simulink model "simulation_Hippocampus_CDC"  (R2021a)
settings: Solver=ode45  StartTime=0.0  StopTime=50  FixedStep=0.00001  MaxStep=0.1  MinStep=0.00001  RelTol=1e-5
libraries: simulink x3
(part 1 of 2)
settings Model: Creator=ch  LastModifiedBy=sf
settings SolverCC: MaxConsecutiveZCs=100000  ZeroCrossAlgorithm=Adaptive  AlgebraicLoopSolver=TrustRegion  PositivePriorityOrder=on  AutoInsertRateTranBlk=on
settings DebuggingCC: MaskedZcDiagnostic=none  IgnoredZcDiagnostic=none  SFMachineParentedDataDiag=warning  ArithmeticOperatorsInVariantConditions=warning
settings SFSimCC: CustomCodeUndefinedFunction=UseInterfaceOnly

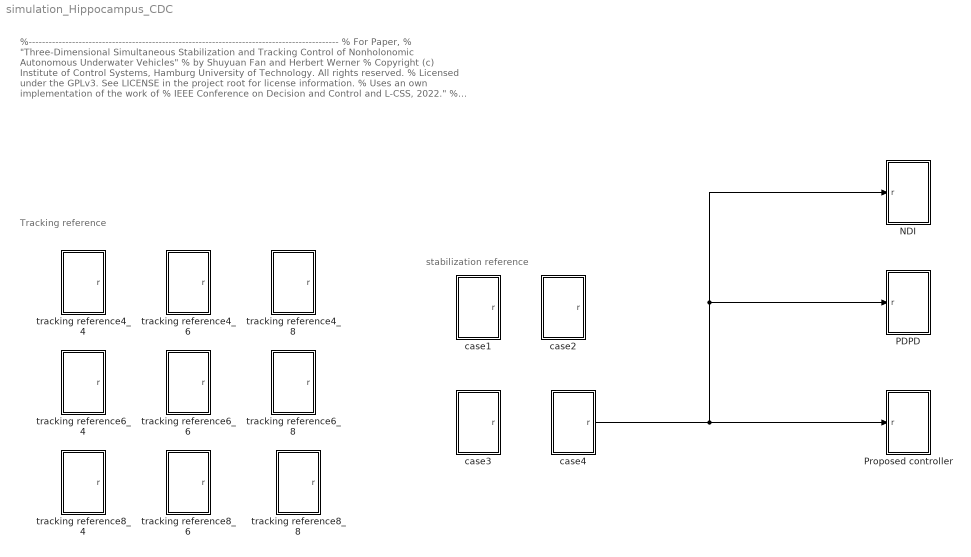
== system simulation_Hippocampus_CDC ==
  note: %---------------------------------------------------------------------------------------------
      | % For Paper,
      | % "Three-Dimensional Simultaneous Stabilization and Tracking Control of Nonholonomic Autonomous Underwater Vehicles"
      | % by Shuyuan Fan and Herbert Werner
      | % Copyright (c) Institute of Control Systems, Hamburg University of Technology. All rights reserved.
      | % Licensed under the GPLv3. See LICENSE in the project root for license information.
      | % Uses an own implementation of the work of
      | % IEEE Conference on Decision and Control and L-CSS, 2022."
      | % Author(s): Shuyuan Fan
      | %--------------------------------------------------------------------------------------------
  note: Tracking reference
  note: stabilization reference
  NDI : Subsystem
  PDPD : Subsystem
  Proposed controller : Subsystem
  case1 : Subsystem
  case2 : Subsystem
  case3 : Subsystem
  case4 : Subsystem
  tracking reference4_4 : Subsystem
  tracking reference4_6 : Subsystem
  tracking reference4_8 : Subsystem
  tracking reference6_4 : Subsystem
  tracking reference6_6 : Subsystem
  tracking reference6_8 : Subsystem
  tracking reference8_4 : Subsystem
  tracking reference8_6 : Subsystem
  tracking reference8_8 : Subsystem
  wires:
  case4/1(r) -> NDI/1(r), PDPD/1(r), Proposed controller/1(r)

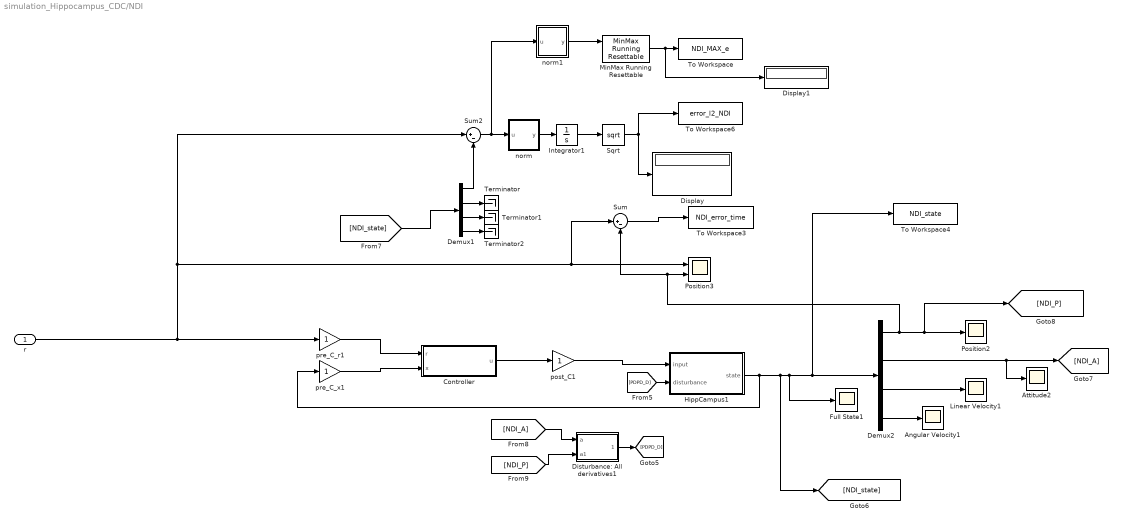
== system simulation_Hippocampus_CDC/NDI ==
  r : Inport
  Angular Velocity1 : Scope
  Attitude2 : Scope
  Controller : Subsystem
  Demux1 : Demux  Outputs=[3 3 3 3]
  Demux2 : Demux  Outputs=[3 3 3 3]
  Display : Display
  Display1 : Display
  Disturbance: All derivatives1 : Subsystem
  Full State1 : Scope
  HippCampus1 : Subsystem
  Integrator1 : Integrator
  Linear Velocity1 : Scope
  MinMax Running Resettable : simulink/Math Operations/MinMax Running Resettable  Function=max  vinit=0.0
  Position2 : Scope
  Position3 : Scope  NumInputPorts=2
  Sqrt : Sqrt  SaturateOnIntegerOverflow=on
  Sum : Sum  Inputs=|+-
  Sum2 : Sum  Inputs=|+-
  Terminator : Terminator
  Terminator1 : Terminator
  Terminator2 : Terminator
  To Workspace : ToWorkspace  VariableName=NDI_MAX_e  SaveFormat=Timeseries  SampleTime=-1
  To Workspace3 : ToWorkspace  VariableName=NDI_error_time  SaveFormat=Timeseries  SampleTime=-1
  To Workspace4 : ToWorkspace  VariableName=NDI_state  SaveFormat=Timeseries  SampleTime=-1
  To Workspace6 : ToWorkspace  VariableName=error_l2_NDI  SaveFormat=Timeseries  SampleTime=-1
      settings: MaxDataPoints=1
  norm : MATLAB Function  TreatAsAtomicUnit=on
  norm1 : MATLAB Function  TreatAsAtomicUnit=on
  post_C1 : Gain
  pre_C_r1 : Gain
  pre_C_x1 : Gain
  wires:
  Controller/1(u) -> post_C1/1
  [PDPD_D] -> HippCampus1/2(disturbance)
  Demux2/2 -> Attitude2/1, [NDI_A]
  HippCampus1/1(state) -> To Workspace4/1, Demux2/1, Full State1/1, [NDI_state], pre_C_x1/1
  pre_C_r1/1 -> Controller/1(r)
  Demux2/3 -> Linear Velocity1/1
  post_C1/1 -> HippCampus1/1(input)
  Disturbance: All derivatives1/1(disturbance) -> [PDPD_D]
  [NDI_P] -> Disturbance: All derivatives1/2(a1)
  pre_C_x1/1 -> Controller/2(x)
  Demux2/4 -> Angular Velocity1/1
  [NDI_A] -> Disturbance: All derivatives1/1(a)
  [NDI_state] -> Demux1/1
  Demux1/3 -> Terminator1/1
  Integrator1/1 -> Sqrt/1
  norm/1(y) -> Integrator1/1
  Demux1/2 -> Terminator/1
  Demux1/1 -> Sum2/2
  Demux1/4 -> Terminator2/1
  Sqrt/1 -> To Workspace6/1, Display/1
  Sum2/1 -> norm1/1(u), norm/1(u)
  norm1/1(y) -> MinMax Running Resettable/1
  MinMax Running Resettable/1 -> Display1/1, To Workspace/1
  Sum/1 -> To Workspace3/1
  r/1 -> Sum/1, Position3/1, Sum2/1, pre_C_r1/1
  Demux2/1 -> [NDI_P], Position2/1, Sum/2, Position3/2

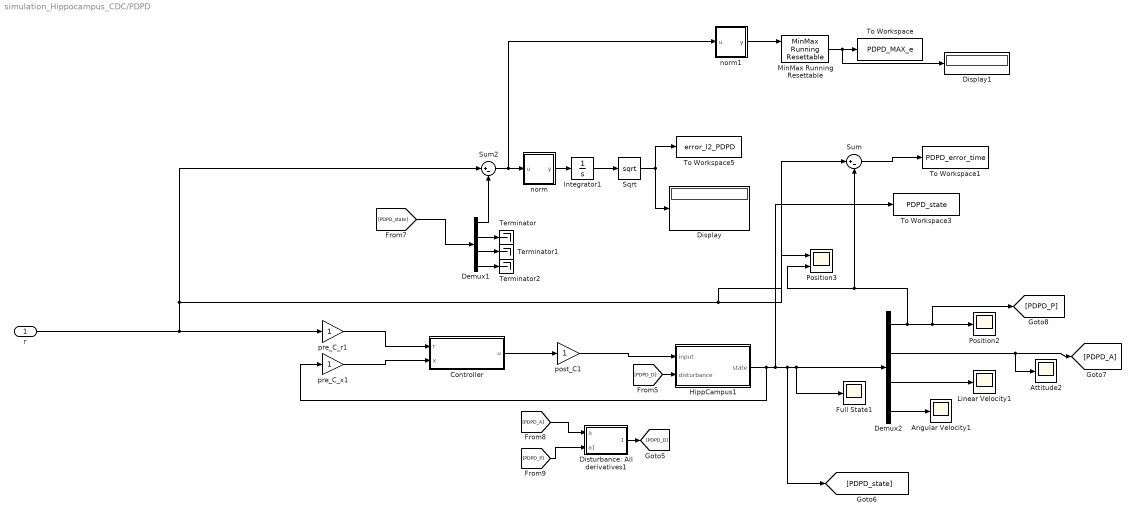
== system simulation_Hippocampus_CDC/PDPD ==
  r : Inport
  Angular Velocity1 : Scope
  Attitude2 : Scope
  Controller : Subsystem
  Demux1 : Demux  Outputs=[3 3 3 3]
  Demux2 : Demux  Outputs=[3 3 3 3]
  Display : Display
  Display1 : Display
  Disturbance: All derivatives1 : Subsystem
  Full State1 : Scope
  HippCampus1 : Subsystem
  Integrator1 : Integrator
  Linear Velocity1 : Scope
  MinMax Running Resettable : simulink/Math Operations/MinMax Running Resettable  Function=max  vinit=0.0
  Position2 : Scope
  Position3 : Scope  NumInputPorts=2
  Sqrt : Sqrt  SaturateOnIntegerOverflow=on
  Sum : Sum  Inputs=|+-
  Sum2 : Sum  Inputs=|+-
  Terminator : Terminator
  Terminator1 : Terminator
  Terminator2 : Terminator
  To Workspace : ToWorkspace  VariableName=PDPD_MAX_e  SaveFormat=Timeseries  SampleTime=-1
  To Workspace1 : ToWorkspace  VariableName=PDPD_error_time  SaveFormat=Timeseries  SampleTime=-1
  To Workspace3 : ToWorkspace  VariableName=PDPD_state  SaveFormat=Timeseries  SampleTime=-1
  To Workspace5 : ToWorkspace  VariableName=error_l2_PDPD  SaveFormat=Timeseries  SampleTime=-1
      settings: MaxDataPoints=1
  norm : MATLAB Function  TreatAsAtomicUnit=on
  norm1 : MATLAB Function  TreatAsAtomicUnit=on
  post_C1 : Gain
  pre_C_r1 : Gain
  pre_C_x1 : Gain
  wires:
  [PDPD_D] -> HippCampus1/2(disturbance)
  Demux2/2 -> Attitude2/1, [PDPD_A]
  HippCampus1/1(state) -> Full State1/1, Demux2/1, [PDPD_state], To Workspace3/1, pre_C_x1/1
  pre_C_r1/1 -> Controller/1(r)
  Demux2/3 -> Linear Velocity1/1
  post_C1/1 -> HippCampus1/1(input)
  Disturbance: All derivatives1/1(disturbance) -> [PDPD_D]
  [PDPD_P] -> Disturbance: All derivatives1/2(a1)
  pre_C_x1/1 -> Controller/2(x)
  Demux2/4 -> Angular Velocity1/1
  [PDPD_A] -> Disturbance: All derivatives1/1(a)
  [PDPD_state] -> Demux1/1
  Demux1/3 -> Terminator1/1
  Integrator1/1 -> Sqrt/1
  norm/1(y) -> Integrator1/1
  Demux1/2 -> Terminator/1
  Demux1/1 -> Sum2/2
  Demux1/4 -> Terminator2/1
  Sqrt/1 -> To Workspace5/1, Display/1
  Controller/1(u) -> post_C1/1
  norm1/1(y) -> MinMax Running Resettable/1
  MinMax Running Resettable/1 -> Display1/1, To Workspace/1
  Sum2/1 -> norm1/1(u), norm/1(u)
  Sum/1 -> To Workspace1/1
  r/1 -> Sum/1, Position3/1, Sum2/1, pre_C_r1/1
  Demux2/1 -> [PDPD_P], Position2/1, Sum/2, Position3/2

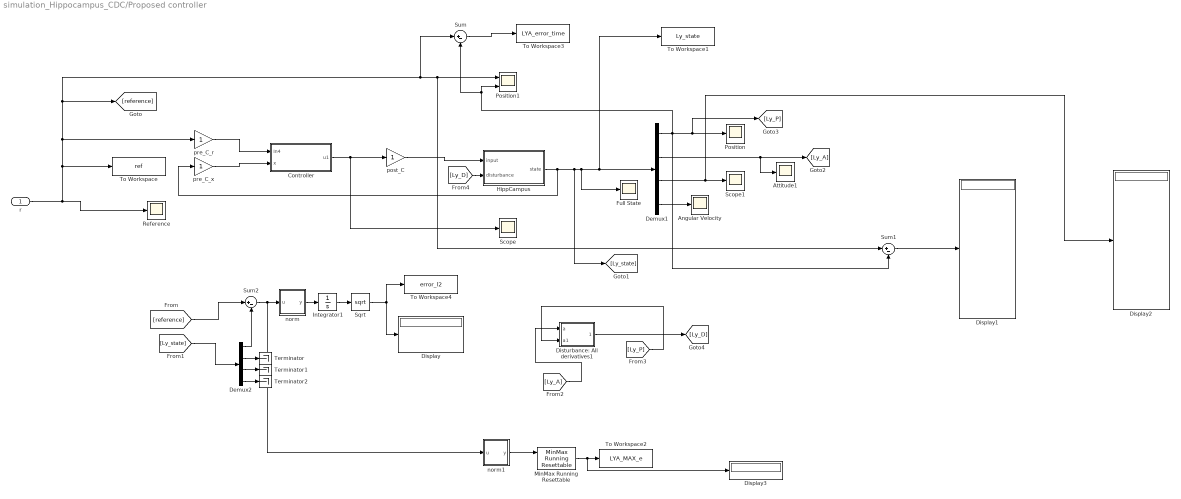
== system simulation_Hippocampus_CDC/Proposed controller ==
  r : Inport
  Angular Velocity : Scope
  Attitude1 : Scope
  Controller : Subsystem
  Demux1 : Demux  Outputs=[3 3 3 3]
  Demux2 : Demux  Outputs=[3 3 3 3]
  Display{,1..3} (4 alike) : Display
  Disturbance: All derivatives1 : Subsystem
  Full State : Scope
  HippCampus : Subsystem
  Integrator1 : Integrator
  MinMax Running Resettable : simulink/Math Operations/MinMax Running Resettable  Function=max  vinit=0.0
  Position : Scope
  Position1 : Scope  NumInputPorts=2
  Reference : Scope
  Scope : Scope
  Scope1 : Scope
  Sqrt : Sqrt  SaturateOnIntegerOverflow=on
  Sum : Sum  Inputs=|+-
  Sum1 : Sum  Inputs=|+-
  Sum2 : Sum  Inputs=|+-
  Terminator : Terminator
  Terminator1 : Terminator
  Terminator2 : Terminator
  To Workspace : ToWorkspace  VariableName=ref  SaveFormat=Timeseries  SampleTime=-1
  To Workspace1 : ToWorkspace  VariableName=Ly_state  SaveFormat=Timeseries  SampleTime=-1
  To Workspace2 : ToWorkspace  VariableName=LYA_MAX_e  SaveFormat=Timeseries  SampleTime=-1
  To Workspace3 : ToWorkspace  VariableName=LYA_error_time  SaveFormat=Timeseries  SampleTime=-1
  To Workspace4 : ToWorkspace  VariableName=error_l2  SaveFormat=Timeseries  SampleTime=-1
      settings: MaxDataPoints=1
  norm : MATLAB Function  TreatAsAtomicUnit=on
  norm1 : MATLAB Function  TreatAsAtomicUnit=on
  post_C : Gain
  pre_C_r : Gain
  pre_C_x : Gain
  wires:
  HippCampus/1(state) -> To Workspace1/1, Demux1/1, Full State/1, [Ly_state], pre_C_x/1
  Disturbance: All derivatives1/1(disturbance) -> [Ly_D]
  Demux1/3 -> Scope1/1, Display2/1
  Demux2/3 -> Terminator1/1
  [Ly_state] -> Demux2/1
  Controller/1(u1) -> Scope/1, post_C/1
  [reference] -> Sum2/1
  Demux2/1 -> Sum2/2
  norm/1(y) -> Integrator1/1
  pre_C_x/1 -> Controller/2(x)
  Integrator1/1 -> Sqrt/1
  Sqrt/1 -> To Workspace4/1, Display/1
  Demux1/4 -> Angular Velocity/1
  [Ly_D] -> HippCampus/2(disturbance)
  Demux1/2 -> Attitude1/1, [Ly_A]
  pre_C_r/1 -> Controller/1(In4)
  Demux2/4 -> Terminator2/1
  Demux1/1 -> [Ly_P], Position/1, Sum/2, Position1/2, Sum1/2
  post_C/1 -> HippCampus/1(input)
  [Ly_P] -> Disturbance: All derivatives1/2(a1)
  Demux2/2 -> Terminator/1
  [Ly_A] -> Disturbance: All derivatives1/1(a)
  Sum2/1 -> norm/1(u), norm1/1(u)
  MinMax Running Resettable/1 -> Display3/1, To Workspace2/1
  norm1/1(y) -> MinMax Running Resettable/1
  Sum/1 -> To Workspace3/1
  r/1 -> Sum/1, Sum1/1, Position1/1, [reference], pre_C_r/1, To Workspace/1, Reference/1
  Sum1/1 -> Display1/1

== system simulation_Hippocampus_CDC/case1 ==
  Constant : Constant  Value=1.5
  Constant1 : Constant
  Constant2 : Constant  Value=2
  Mux3 : Mux  Inputs=[1 1 1]
  r : Outport
  wires:
  Constant1/1 -> Mux3/3
  Constant2/1 -> Mux3/1
  Constant/1 -> Mux3/2
  Mux3/1 -> r/1  "r"

== system simulation_Hippocampus_CDC/case2 ==
  Constant : Constant  Value=-1.5
  Constant1 : Constant  Value=-1
  Constant2 : Constant  Value=2
  Mux3 : Mux  Inputs=[1 1 1]
  r : Outport
  wires:
  Constant1/1 -> Mux3/3
  Constant2/1 -> Mux3/1
  Constant/1 -> Mux3/2
  Mux3/1 -> r/1  "r"

== system simulation_Hippocampus_CDC/case3 ==
  Constant : Constant  Value=2
  Constant1 : Constant  Value=-1
  Constant2 : Constant  Value=1.5
  Mux3 : Mux  Inputs=[1 1 1]
  r : Outport
  wires:
  Constant1/1 -> Mux3/3
  Constant2/1 -> Mux3/1
  Constant/1 -> Mux3/2
  Mux3/1 -> r/1  "r"

== system simulation_Hippocampus_CDC/case4 ==
  Constant : Constant  Value=-2
  Constant1 : Constant  Value=1.5
  Constant2 : Constant
  Mux3 : Mux  Inputs=[1 1 1]
  r : Outport
  wires:
  Constant1/1 -> Mux3/3
  Constant2/1 -> Mux3/1
  Constant/1 -> Mux3/2
  Mux3/1 -> r/1  "r"

== system simulation_Hippocampus_CDC/tracking reference4_4 ==
  Clock : Clock
  Cos : Trigonometry
  Cos1 : Trigonometry
  Gain5 : Gain  Gain=0.1
  Gain6 : Gain  Gain=4
  Gain7 : Gain  Gain=4
  Gain8 : Gain  Gain=pi/15
  Gain9 : Gain  Gain=pi/30
  Mux : Mux  Inputs=3
  r : Outport
  wires:
  Gain9/1 -> Cos/1
  Gain6/1 -> Mux/1
  Gain7/1 -> Mux/2
  Cos1/1 -> Gain6/1
  Cos/1 -> Gain7/1
  Mux/1 -> r/1  "r"
  Gain8/1 -> Cos1/1
  Gain5/1 -> Mux/3
  Clock/1 -> Gain5/1, Gain9/1, Gain8/1

== system simulation_Hippocampus_CDC/tracking reference4_6 ==
  Clock : Clock
  Cos : Trigonometry
  Cos1 : Trigonometry
  Gain5 : Gain  Gain=0.1
  Gain6 : Gain  Gain=4
  Gain7 : Gain  Gain=6
  Gain8 : Gain  Gain=pi/15
  Gain9 : Gain  Gain=pi/30
  Mux : Mux  Inputs=3
  r : Outport
  wires:
  Gain9/1 -> Cos/1
  Gain6/1 -> Mux/1
  Gain7/1 -> Mux/2
  Cos1/1 -> Gain6/1
  Cos/1 -> Gain7/1
  Mux/1 -> r/1  "r"
  Gain8/1 -> Cos1/1
  Gain5/1 -> Mux/3
  Clock/1 -> Gain5/1, Gain9/1, Gain8/1

== system simulation_Hippocampus_CDC/tracking reference4_8 ==
  Clock : Clock
  Cos : Trigonometry
  Cos1 : Trigonometry
  Gain5 : Gain  Gain=0.1
  Gain6 : Gain  Gain=4
  Gain7 : Gain  Gain=8
  Gain8 : Gain  Gain=pi/15
  Gain9 : Gain  Gain=pi/30
  Mux : Mux  Inputs=3
  r : Outport
  wires:
  Gain9/1 -> Cos/1
  Gain6/1 -> Mux/1
  Gain7/1 -> Mux/2
  Cos1/1 -> Gain6/1
  Cos/1 -> Gain7/1
  Mux/1 -> r/1  "r"
  Gain8/1 -> Cos1/1
  Gain5/1 -> Mux/3
  Clock/1 -> Gain5/1, Gain9/1, Gain8/1

== system simulation_Hippocampus_CDC/tracking reference6_4 ==
  Clock : Clock
  Cos : Trigonometry
  Cos1 : Trigonometry
  Gain5 : Gain  Gain=0.1
  Gain6 : Gain  Gain=6
  Gain7 : Gain  Gain=4
  Gain8 : Gain  Gain=pi/15
  Gain9 : Gain  Gain=pi/30
  Mux : Mux  Inputs=3
  r : Outport
  wires:
  Gain9/1 -> Cos/1
  Gain6/1 -> Mux/1
  Gain7/1 -> Mux/2
  Cos1/1 -> Gain6/1
  Cos/1 -> Gain7/1
  Mux/1 -> r/1  "r"
  Gain8/1 -> Cos1/1
  Gain5/1 -> Mux/3
  Clock/1 -> Gain5/1, Gain9/1, Gain8/1

== system simulation_Hippocampus_CDC/tracking reference6_6 ==
  Clock : Clock
  Cos : Trigonometry
  Cos1 : Trigonometry
  Gain5 : Gain  Gain=0.1
  Gain6 : Gain  Gain=6
  Gain7 : Gain  Gain=6
  Gain8 : Gain  Gain=pi/15
  Gain9 : Gain  Gain=pi/30
  Mux : Mux  Inputs=3
  r : Outport
  wires:
  Gain9/1 -> Cos/1
  Gain6/1 -> Mux/1
  Gain7/1 -> Mux/2
  Cos1/1 -> Gain6/1
  Cos/1 -> Gain7/1
  Mux/1 -> r/1  "r"
  Gain8/1 -> Cos1/1
  Gain5/1 -> Mux/3
  Clock/1 -> Gain5/1, Gain9/1, Gain8/1

== system simulation_Hippocampus_CDC/tracking reference6_8 ==
  Clock : Clock
  Cos : Trigonometry
  Cos1 : Trigonometry
  Gain5 : Gain  Gain=0.1
  Gain6 : Gain  Gain=6
  Gain7 : Gain  Gain=8
  Gain8 : Gain  Gain=pi/15
  Gain9 : Gain  Gain=pi/30
  Mux : Mux  Inputs=3
  r : Outport
  wires:
  Gain9/1 -> Cos/1
  Gain6/1 -> Mux/1
  Gain7/1 -> Mux/2
  Cos1/1 -> Gain6/1
  Cos/1 -> Gain7/1
  Mux/1 -> r/1  "r"
  Gain8/1 -> Cos1/1
  Gain5/1 -> Mux/3
  Clock/1 -> Gain5/1, Gain9/1, Gain8/1

== system simulation_Hippocampus_CDC/tracking reference8_4 ==
  Clock : Clock
  Cos : Trigonometry
  Cos1 : Trigonometry
  Gain5 : Gain  Gain=0.1
  Gain6 : Gain  Gain=8
  Gain7 : Gain  Gain=4
  Gain8 : Gain  Gain=pi/15
  Gain9 : Gain  Gain=pi/30
  Mux : Mux  Inputs=3
  r : Outport
  wires:
  Gain9/1 -> Cos/1
  Gain6/1 -> Mux/1
  Gain7/1 -> Mux/2
  Cos1/1 -> Gain6/1
  Cos/1 -> Gain7/1
  Mux/1 -> r/1  "r"
  Gain8/1 -> Cos1/1
  Gain5/1 -> Mux/3
  Clock/1 -> Gain5/1, Gain9/1, Gain8/1

== system simulation_Hippocampus_CDC/tracking reference8_6 ==
  Clock : Clock
  Cos : Trigonometry
  Cos1 : Trigonometry
  Gain5 : Gain  Gain=0.1
  Gain6 : Gain  Gain=8
  Gain7 : Gain  Gain=6
  Gain8 : Gain  Gain=pi/15
  Gain9 : Gain  Gain=pi/30
  Mux : Mux  Inputs=3
  r : Outport
  wires:
  Gain9/1 -> Cos/1
  Gain6/1 -> Mux/1
  Gain7/1 -> Mux/2
  Cos1/1 -> Gain6/1
  Cos/1 -> Gain7/1
  Mux/1 -> r/1  "r"
  Gain8/1 -> Cos1/1
  Gain5/1 -> Mux/3
  Clock/1 -> Gain5/1, Gain9/1, Gain8/1

== system simulation_Hippocampus_CDC/tracking reference8_8 ==
  Clock : Clock
  Cos : Trigonometry
  Cos1 : Trigonometry
  Gain5 : Gain  Gain=0.1
  Gain6 : Gain  Gain=8
  Gain7 : Gain  Gain=8
  Gain8 : Gain  Gain=pi/15
  Gain9 : Gain  Gain=pi/30
  Mux : Mux  Inputs=3
  r : Outport
  wires:
  Gain9/1 -> Cos/1
  Gain6/1 -> Mux/1
  Gain7/1 -> Mux/2
  Cos1/1 -> Gain6/1
  Cos/1 -> Gain7/1
  Mux/1 -> r/1  "r"
  Gain8/1 -> Cos1/1
  Gain5/1 -> Mux/3
  Clock/1 -> Gain5/1, Gain9/1, Gain8/1

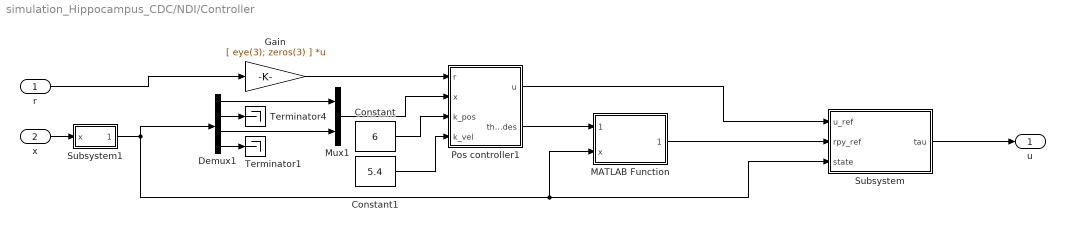
== system simulation_Hippocampus_CDC/NDI/Controller ==
  r : Inport
  x : Inport  Port=2
  Constant : Constant  Value=6
  Constant1 : Constant  Value=5.4
  Demux1 : Demux  Outputs=[3 3 3 3]
  Gain : Gain  Gain=[ eye(3); zeros(3) ]  Multiplication=Matrix(K*u) (u vector)
  MATLAB Function : MATLAB Function  TreatAsAtomicUnit=on
  Mux1 : Mux  Inputs=2
  Pos controller1 : MATLAB Function  TreatAsAtomicUnit=on
  Subsystem : Subsystem
  Subsystem1 : Subsystem
  Terminator1 : Terminator
  Terminator4 : Terminator
  u : Outport
  wires:
  Subsystem/1(tau) -> u/1
  Constant/1 -> Pos controller1/3(k_pos)
  r/1 -> Gain/1
  Constant1/1 -> Pos controller1/4(k_vel)
  Demux1/3 -> Mux1/2
  Subsystem1/1(x_2pi) -> Demux1/1, MATLAB Function/2(x), Subsystem/3(state)
  Mux1/1 -> Pos controller1/2(x)
  Gain/1 -> Pos controller1/1(r)
  Demux1/1 -> Mux1/1
  Pos controller1/1(u) -> Subsystem/1(u_ref)
  Pos controller1/2(theta_des) -> MATLAB Function/1("theta_des ")
  Demux1/2 -> Terminator4/1
  Demux1/4 -> Terminator1/1
  x/1 -> Subsystem1/1(x)
  MATLAB Function/1(theta_des) -> Subsystem/2(rpy_ref)

== system simulation_Hippocampus_CDC/NDI/Disturbance: All derivatives1 ==
  a : Inport
  a1 : Inport  Port=2
  Gain1 : Gain  Gain=0  Multiplication=Matrix(K*u)
  Gain2 : Gain  Gain=0  Multiplication=Matrix(K*u)
  Gain3 : Gain  Gain=0  Multiplication=Matrix(K*u)
  Sum2 : Sum  Inputs=|+++
  disturbance2 : Subsystem
  disturbance3 : Subsystem
  old disturbance : Subsystem
  disturbance : Outport
  wires:
  Sum2/1 -> disturbance/1
  Gain1/1 -> Sum2/1
  disturbance2/1(Out1) -> Gain2/1
  a/1 -> disturbance3/1(a)
  a1/1 -> disturbance3/2(a1)
  disturbance3/1(d) -> Gain1/1
  Gain2/1 -> Sum2/2
  old disturbance/1(Out1) -> Gain3/1
  Gain3/1 -> Sum2/3

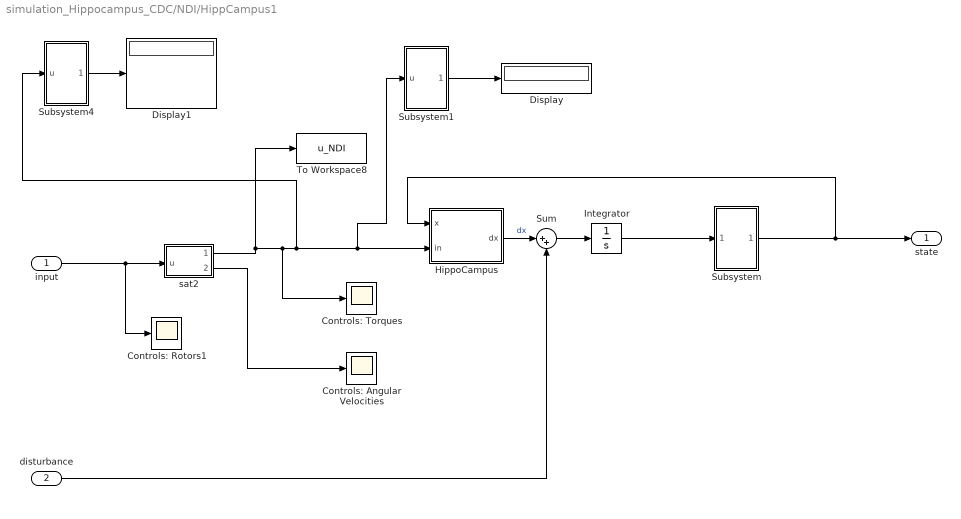
== system simulation_Hippocampus_CDC/NDI/HippCampus1 ==
  input : Inport
  disturbance : Inport  Port=2
  Controls: Angular Velocities : Scope
  Controls: Rotors1 : Scope
  Controls: Torques : Scope
  Display : Display
  Display1 : Display
  HippoCampus : MATLAB Function  TreatAsAtomicUnit=on
  Integrator : Integrator  InitialCondition=[0; 0; 0; 0;0;0;zeros(6,1)]
  Subsystem : Subsystem
  Subsystem1 : Subsystem
  Subsystem4 : Subsystem
  Sum : Sum  Inputs=|++
  To Workspace8 : ToWorkspace  VariableName=u_NDI  SaveFormat=Timeseries  SampleTime=-1
  sat2 : MATLAB Function  TreatAsAtomicUnit=on
  state : Outport
  wires:
  HippoCampus/1(dx) -> Sum/1  "dx"
  Sum/1 -> Integrator/1
  sat2/2(omega) -> Controls: Angular Velocities/1
  input/1 -> sat2/1(u), Controls: Rotors1/1
  disturbance/1 -> Sum/2
  Integrator/1 -> Subsystem/1(In1)
  Subsystem/1(state) -> state/1, HippoCampus/1(x)
  sat2/1(u_sat) -> To Workspace8/1, Subsystem4/1(u), Subsystem1/1(u), HippoCampus/2(in), Controls: Torques/1
  Subsystem4/1(Out1) -> Display1/1
  Subsystem1/1(Out1) -> Display/1

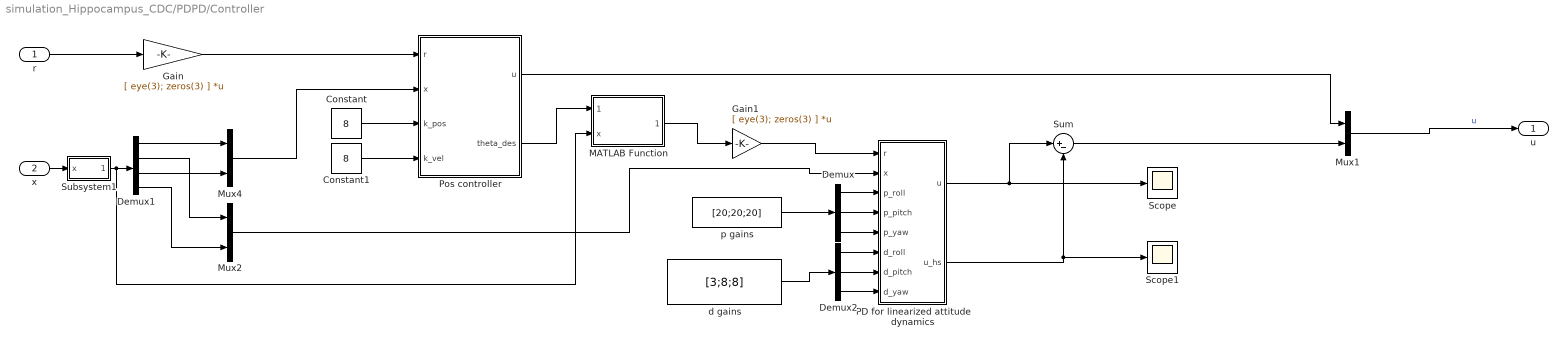
== system simulation_Hippocampus_CDC/PDPD/Controller ==
  r : Inport
  x : Inport  Port=2
  Constant : Constant  Value=8
  Constant1 : Constant  Value=8
  Demux : Demux  Outputs=3
  Demux1 : Demux  Outputs=[3 3 3 3]
  Demux2 : Demux  Outputs=3
  Gain : Gain  Gain=[ eye(3); zeros(3) ]  Multiplication=Matrix(K*u) (u vector)
  Gain1 : Gain  Gain=[ eye(3); zeros(3) ]  Multiplication=Matrix(K*u) (u vector)
  MATLAB Function : MATLAB Function  TreatAsAtomicUnit=on
  Mux1 : Mux  Inputs=2
  Mux2 : Mux  Inputs=2
  Mux4 : Mux  Inputs=2
  PD for linearized attitude dynamics : MATLAB Function  TreatAsAtomicUnit=on
  Pos controller : MATLAB Function  TreatAsAtomicUnit=on
  Scope : Scope
  Scope1 : Scope
  Subsystem1 : Subsystem
  Sum : Sum  Inputs=|+-
  d gains : Constant  Value=[3;8;8]
  p gains : Constant  Value=[20;20;20]
  u : Outport
  wires:
  Mux1/1 -> u/1  "u"
  Pos controller/1(u) -> Mux1/1
  x/1 -> Subsystem1/1(x)
  Demux1/1 -> Mux4/1
  Demux1/3 -> Mux4/2
  Mux4/1 -> Pos controller/2(x)
  Demux1/2 -> Mux2/1
  Demux1/4 -> Mux2/2
  Mux2/1 -> PD for linearized attitude dynamics/2(x)
  Pos controller/2(theta_des) -> MATLAB Function/1("theta_des ")
  Gain1/1 -> PD for linearized attitude dynamics/1(r)
  PD for linearized attitude dynamics/2(u_hs) -> Sum/2, Scope1/1
  PD for linearized attitude dynamics/1(u) -> Sum/1, Scope/1
  Sum/1 -> Mux1/2
  r/1 -> Gain/1
  Gain/1 -> Pos controller/1(r)
  Constant/1 -> Pos controller/3(k_pos)
  Constant1/1 -> Pos controller/4(k_vel)
  p gains/1 -> Demux/1
  Demux/1 -> PD for linearized attitude dynamics/3(p_roll)
  Demux/2 -> PD for linearized attitude dynamics/4(p_pitch)
  Demux/3 -> PD for linearized attitude dynamics/5(p_yaw)
  d gains/1 -> Demux2/1
  Demux2/1 -> PD for linearized attitude dynamics/6(d_roll)
  Demux2/2 -> PD for linearized attitude dynamics/7(d_pitch)
  Demux2/3 -> PD for linearized attitude dynamics/8(d_yaw)
  MATLAB Function/1(theta_des) -> Gain1/1
  Subsystem1/1(x_2pi) -> MATLAB Function/2(x), Demux1/1

== system simulation_Hippocampus_CDC/PDPD/Disturbance: All derivatives1 ==
  a : Inport
  a1 : Inport  Port=2
  Gain1 : Gain  Gain=0  Multiplication=Matrix(K*u)
  Gain2 : Gain  Gain=0  Multiplication=Matrix(K*u)
  Gain3 : Gain  Gain=0  Multiplication=Matrix(K*u)
  Sum2 : Sum  Inputs=|+++
  disturbance2 : Subsystem
  disturbance3 : Subsystem
  old disturbance : Subsystem
  disturbance : Outport
  wires:
  Sum2/1 -> disturbance/1
  Gain1/1 -> Sum2/1
  disturbance2/1(Out1) -> Gain2/1
  a/1 -> disturbance3/1(a)
  a1/1 -> disturbance3/2(a1)
  disturbance3/1(d) -> Gain1/1
  Gain2/1 -> Sum2/2
  old disturbance/1(Out1) -> Gain3/1
  Gain3/1 -> Sum2/3

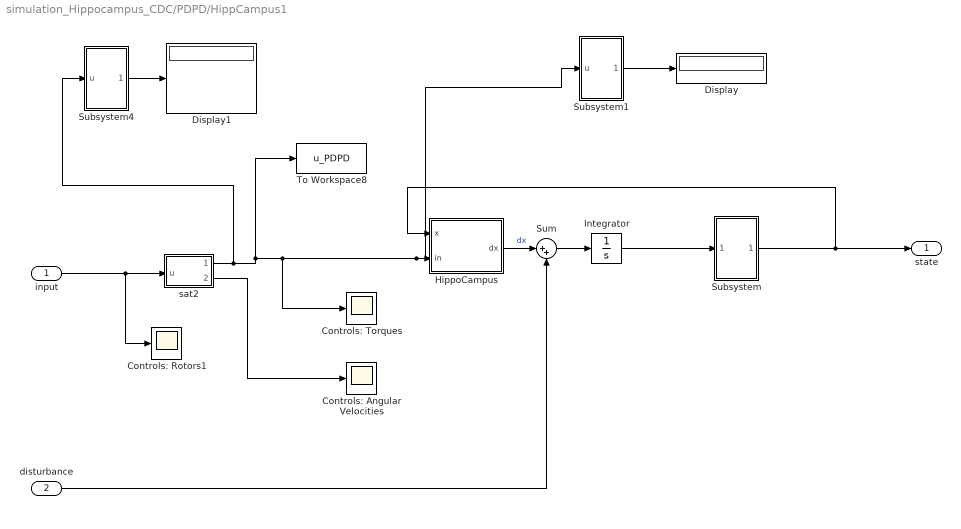
== system simulation_Hippocampus_CDC/PDPD/HippCampus1 ==
  input : Inport
  disturbance : Inport  Port=2
  Controls: Angular Velocities : Scope
  Controls: Rotors1 : Scope
  Controls: Torques : Scope
  Display : Display
  Display1 : Display
  HippoCampus : MATLAB Function  TreatAsAtomicUnit=on
  Integrator : Integrator  InitialCondition=[0; 0; 0; 0;0;0;zeros(6,1)]
  Subsystem : Subsystem
  Subsystem1 : Subsystem
  Subsystem4 : Subsystem
  Sum : Sum  Inputs=|++
  To Workspace8 : ToWorkspace  VariableName=u_PDPD  SaveFormat=Timeseries  SampleTime=-1
  sat2 : MATLAB Function  TreatAsAtomicUnit=on
  state : Outport
  wires:
  HippoCampus/1(dx) -> Sum/1  "dx"
  Sum/1 -> Integrator/1
  sat2/2(omega) -> Controls: Angular Velocities/1
  input/1 -> sat2/1(u), Controls: Rotors1/1
  disturbance/1 -> Sum/2
  Integrator/1 -> Subsystem/1(In1)
  Subsystem/1(state) -> state/1, HippoCampus/1(x)
  Subsystem4/1(Out1) -> Display1/1
  Subsystem1/1(Out1) -> Display/1
  sat2/1(u_sat) -> Subsystem4/1(u), To Workspace8/1, Subsystem1/1(u), HippoCampus/2(in), Controls: Torques/1

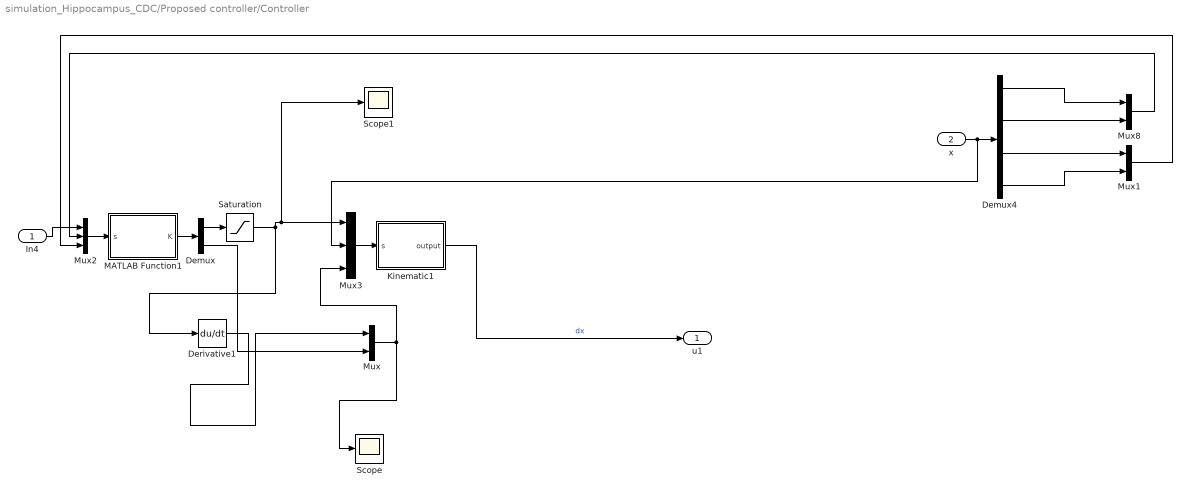
== system simulation_Hippocampus_CDC/Proposed controller/Controller ==
  In4 : Inport
  x : Inport  Port=2
  Demux : Demux  Outputs=[4 4]
  Demux4 : Demux  Outputs=[3 3 3 3]
  Derivative1 : Derivative  CoefficientInTFapproximation=1
  Kinematic1 : MATLAB Function  TreatAsAtomicUnit=on
  MATLAB Function1 : MATLAB Function  TreatAsAtomicUnit=on
  Mux : Mux  Inputs=2
  Mux1 : Mux  Inputs=2
  Mux2 : Mux  Inputs=3
  Mux3 : Mux  Inputs=3
  Mux8 : Mux  Inputs=2
  Saturation : Saturate  UpperLimit=[5;5;5;5]  LowerLimit=-[10;10;10;10]
  Scope : Scope
  Scope1 : Scope
  u1 : Outport
  wires:
  Demux4/2 -> Mux8/2
  Demux4/1 -> Mux8/1
  x/1 -> Mux3/2, Demux4/1
  Demux4/3 -> Mux1/1
  Demux4/4 -> Mux1/2
  Kinematic1/1(output) -> u1/1  "dx"
  Mux2/1 -> MATLAB Function1/1(s)
  Mux3/1 -> Kinematic1/1(s)
  In4/1 -> Mux2/1
  Mux1/1 -> Mux2/3
  Mux8/1 -> Mux2/2
  MATLAB Function1/1(K) -> Demux/1
  Demux/2 -> Mux/2
  Mux/1 -> Mux3/3, Scope/1
  Demux/1 -> Saturation/1
  Derivative1/1 -> Mux/1
  Saturation/1 -> Derivative1/1, Mux3/1, Scope1/1

== system simulation_Hippocampus_CDC/Proposed controller/Disturbance: All derivatives1 ==
  a : Inport
  a1 : Inport  Port=2
  Gain1 : Gain  Gain=0  Multiplication=Matrix(K*u)
  Gain2 : Gain  Gain=0  Multiplication=Matrix(K*u)
  Gain3 : Gain  Gain=0  Multiplication=Matrix(K*u)
  Sum2 : Sum  Inputs=|+++
  disturbance2 : Subsystem
  disturbance3 : Subsystem
  old disturbance : Subsystem
  disturbance : Outport
  wires:
  Sum2/1 -> disturbance/1
  Gain1/1 -> Sum2/1
  disturbance2/1(Out1) -> Gain2/1
  a/1 -> disturbance3/1(a)
  a1/1 -> disturbance3/2(a1)
  disturbance3/1(d) -> Gain1/1
  Gain2/1 -> Sum2/2
  old disturbance/1(Out1) -> Gain3/1
  Gain3/1 -> Sum2/3

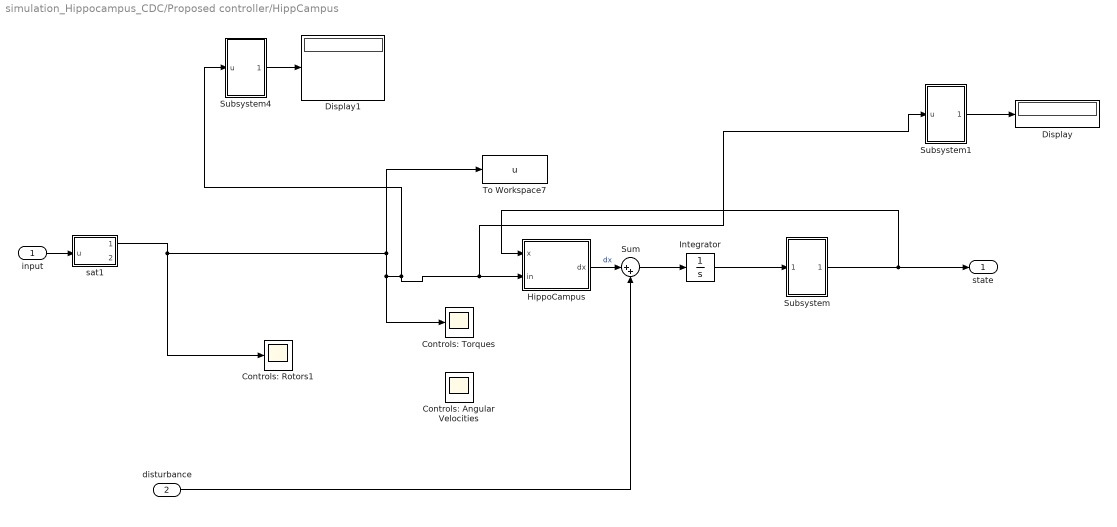
== system simulation_Hippocampus_CDC/Proposed controller/HippCampus ==
  input : Inport
  disturbance : Inport  Port=2
  Controls: Angular Velocities : Scope
  Controls: Rotors1 : Scope
  Controls: Torques : Scope
  Display : Display
  Display1 : Display
  HippoCampus : MATLAB Function  TreatAsAtomicUnit=on
  Integrator : Integrator  InitialCondition=[0; 0; 0; 0;0;0;zeros(6,1)]
  Subsystem : Subsystem
  Subsystem1 : Subsystem
  Subsystem4 : Subsystem
  Sum : Sum  Inputs=|++
  To Workspace7 : ToWorkspace  VariableName=u  SaveFormat=Timeseries  SampleTime=-1
  sat1 : MATLAB Function  TreatAsAtomicUnit=on
  state : Outport
  wires:
  HippoCampus/1(dx) -> Sum/1  "dx"
  Sum/1 -> Integrator/1
  ? -> Controls: Angular Velocities/1
  disturbance/1 -> Sum/2
  Integrator/1 -> Subsystem/1(In1)
  Subsystem/1(state) -> state/1, HippoCampus/1(x)
  Subsystem4/1(Out1) -> Display1/1
  Subsystem1/1(Out1) -> Display/1
  sat1/1(u_sat) -> Controls: Rotors1/1, Controls: Torques/1, Subsystem1/1(u), HippoCampus/2(in), Subsystem4/1(u), To Workspace7/1
  input/1 -> sat1/1(u)

== system simulation_Hippocampus_CDC/NDI/Controller/Subsystem ==
  u_ref : Inport
  rpy_ref : Inport  Port=2
  state : Inport  Port=3
  Demux : Demux
  Manual Switch : ManualSwitch
  Mux : Mux  Inputs=2
  Mux1 : Mux
  Subsystem1 : Subsystem
  Subsystem2 : Subsystem
  Terminator : Terminator
  tau : Outport
  wires:
  state/1 -> Subsystem1/2(state), Subsystem2/1(state)
  Subsystem1/1(pqr_ref) -> Mux/2
  Subsystem2/1(tau) -> Manual Switch/2, Demux/1
  rpy_ref/1 -> Subsystem1/1(rpy_ref)
  Mux/1 -> Subsystem2/2(upqr_ref)
  u_ref/1 -> Mux1/1, Mux/1
  Demux/2 -> Mux1/2
  Demux/3 -> Mux1/3
  Demux/4 -> Mux1/4
  Manual Switch/1 -> tau/1
  Mux1/1 -> Manual Switch/1
  Demux/1 -> Terminator/1

== system simulation_Hippocampus_CDC/NDI/Controller/Subsystem1 ==
  x : Inport
  Demux1 : Demux  Outputs=12
  MATLAB Function : MATLAB Function  TreatAsAtomicUnit=on
  Mux1 : Mux  Inputs=12
  x_2pi : Outport
  wires:
  Mux1/1 -> x_2pi/1
  x/1 -> Demux1/1
  Demux1/6 -> MATLAB Function/1(u)
  Demux1/1 -> Mux1/1
  Demux1/2 -> Mux1/2
  Demux1/3 -> Mux1/3
  Demux1/4 -> Mux1/4
  Demux1/5 -> Mux1/5
  Demux1/7 -> Mux1/7
  Demux1/8 -> Mux1/8
  Demux1/9 -> Mux1/9
  Demux1/10 -> Mux1/10
  Demux1/11 -> Mux1/11
  Demux1/12 -> Mux1/12
  MATLAB Function/1(y) -> Mux1/6

== system simulation_Hippocampus_CDC/NDI/Disturbance: All derivatives1/disturbance2 ==
  Gain : Gain  Gain=[zeros(6,1);ones(6,1)]  Multiplication=Matrix(K*u)
  Step2 : Step  Time=50  After=0.5  SampleTime=0
  Step3 : Step  Time=55  After=-0.5  SampleTime=0
  Sum1 : Sum  Inputs=|++
  Out1 : Outport
  wires:
  Step2/1 -> Sum1/1
  Step3/1 -> Sum1/2
  Gain/1 -> Out1/1
  Sum1/1 -> Gain/1

== system simulation_Hippocampus_CDC/NDI/Disturbance: All derivatives1/disturbance3 ==
  a : Inport
  a1 : Inport  Port=2
  Constant : Constant  Value=10
  MATLAB Function : MATLAB Function  TreatAsAtomicUnit=on
  Subsystem : Subsystem
  Subsystem1 : Subsystem
  d : Outport
  wires:
  Subsystem1/1(Out1) -> MATLAB Function/3(u_wave)
  Constant/1 -> MATLAB Function/5(u_un)
  Subsystem/1(Out1) -> MATLAB Function/4(u_c)
  MATLAB Function/1(d) -> d/1
  a1/1 -> MATLAB Function/1(p)
  a/1 -> MATLAB Function/2(a)

== system simulation_Hippocampus_CDC/NDI/Disturbance: All derivatives1/old disturbance ==
  Gain : Gain  Gain=ones(12,1)  Multiplication=Matrix(K*u)
  Step : Step  Time=50  After=0.5  SampleTime=0
  Step1 : Step  Time=55  After=-0.5  SampleTime=0
  Step2 : Step  Time=100  After=0.5  SampleTime=0
  Step3 : Step  Time=105  After=-0.5  SampleTime=0
  Sum : Sum  Inputs=|++
  Sum2 : Sum  Inputs=|++
  Sum3 : Sum  Inputs=|++
  Out1 : Outport
  wires:
  Gain/1 -> Out1/1
  Sum3/1 -> Gain/1
  Step3/1 -> Sum2/2
  Step/1 -> Sum/1
  Step1/1 -> Sum/2
  Step2/1 -> Sum2/1
  Sum/1 -> Sum3/1
  Sum2/1 -> Sum3/2

== system simulation_Hippocampus_CDC/NDI/HippCampus1/Subsystem ==
  In1 : Inport
  Demux : Demux  Outputs=[5 1 6]
  MATLAB Function : MATLAB Function  TreatAsAtomicUnit=on
  Mux : Mux  Inputs=3
  state : Outport
  wires:
  Demux/2 -> MATLAB Function/1(u)
  MATLAB Function/1(y) -> Mux/2
  In1/1 -> Demux/1
  Demux/3 -> Mux/3
  Demux/1 -> Mux/1
  Mux/1 -> state/1

== system simulation_Hippocampus_CDC/NDI/HippCampus1/Subsystem1 ==
  u : Inport
  Integrator2 : Integrator
  Sqrt1 : Sqrt  SaturateOnIntegerOverflow=on
  norm1 : MATLAB Function  TreatAsAtomicUnit=on
  Out1 : Outport
  wires:
  norm1/1(y) -> Integrator2/1
  Sqrt1/1 -> Out1/1
  Integrator2/1 -> Sqrt1/1
  u/1 -> norm1/1(u)

== system simulation_Hippocampus_CDC/NDI/HippCampus1/Subsystem4 ==
  u : Inport
  Demux : Demux
  Mux : Mux
  Subsystem : Subsystem
  Subsystem1 : Subsystem
  Subsystem2 : Subsystem
  Subsystem3 : Subsystem
  Out1 : Outport
  wires:
  Subsystem2/1(Out1) -> Mux/3
  Demux/4 -> Subsystem3/1(u)
  Demux/3 -> Subsystem2/1(u)
  Subsystem1/1(Out1) -> Mux/2
  Demux/2 -> Subsystem1/1(u)
  Subsystem3/1(Out1) -> Mux/4
  Demux/1 -> Subsystem/1(u)
  Subsystem/1(Out1) -> Mux/1
  Mux/1 -> Out1/1
  u/1 -> Demux/1

== system simulation_Hippocampus_CDC/PDPD/Controller/Subsystem1 ==
  x : Inport
  Demux1 : Demux  Outputs=12
  MATLAB Function : MATLAB Function  TreatAsAtomicUnit=on
  Mux1 : Mux  Inputs=12
  x_2pi : Outport
  wires:
  Mux1/1 -> x_2pi/1
  x/1 -> Demux1/1
  Demux1/6 -> MATLAB Function/1(u)
  Demux1/1 -> Mux1/1
  Demux1/2 -> Mux1/2
  Demux1/3 -> Mux1/3
  Demux1/4 -> Mux1/4
  Demux1/5 -> Mux1/5
  Demux1/7 -> Mux1/7
  Demux1/8 -> Mux1/8
  Demux1/9 -> Mux1/9
  Demux1/10 -> Mux1/10
  Demux1/11 -> Mux1/11
  Demux1/12 -> Mux1/12
  MATLAB Function/1(y) -> Mux1/6

== system simulation_Hippocampus_CDC/PDPD/Disturbance: All derivatives1/disturbance2 ==
  Gain : Gain  Gain=[zeros(6,1);ones(6,1)]  Multiplication=Matrix(K*u)
  Step2 : Step  Time=50  After=0.5  SampleTime=0
  Step3 : Step  Time=55  After=-0.5  SampleTime=0
  Sum1 : Sum  Inputs=|++
  Out1 : Outport
  wires:
  Step2/1 -> Sum1/1
  Step3/1 -> Sum1/2
  Gain/1 -> Out1/1
  Sum1/1 -> Gain/1

== system simulation_Hippocampus_CDC/PDPD/Disturbance: All derivatives1/disturbance3 ==
  note: Subsystem
  a : Inport
  a1 : Inport  Port=2
  Constant : Constant  Value=10
  Constant2 : Constant  Value=10
  Constant3 : Constant  Value=45
  Constant4 : Constant  Value=20
  Gain : Gain  Gain=pi/180
  Gain1 : Gain  Gain=pi/180
  MATLAB Function : MATLAB Function  TreatAsAtomicUnit=on
  Mux : Mux  Inputs=3
  Subsystem1 : Subsystem
  d : Outport
  wires:
  Subsystem1/1(Out1) -> MATLAB Function/3(u_wave)
  Constant/1 -> MATLAB Function/5(u_un)
  Mux/1 -> MATLAB Function/4(u_c)
  MATLAB Function/1(d) -> d/1
  a1/1 -> MATLAB Function/1(p)
  a/1 -> MATLAB Function/2(a)
  Constant4/1 -> Mux/1
  Gain/1 -> Mux/2
  Gain1/1 -> Mux/3
  Constant3/1 -> Gain1/1
  Constant2/1 -> Gain/1

== system simulation_Hippocampus_CDC/PDPD/Disturbance: All derivatives1/old disturbance ==
  Gain : Gain  Gain=ones(12,1)  Multiplication=Matrix(K*u)
  Step : Step  Time=50  After=0.5  SampleTime=0
  Step1 : Step  Time=55  After=-0.5  SampleTime=0
  Step2 : Step  Time=100  After=0.5  SampleTime=0
  Step3 : Step  Time=105  After=-0.5  SampleTime=0
  Sum : Sum  Inputs=|++
  Sum2 : Sum  Inputs=|++
  Sum3 : Sum  Inputs=|++
  Out1 : Outport
  wires:
  Gain/1 -> Out1/1
  Sum3/1 -> Gain/1
  Step3/1 -> Sum2/2
  Step/1 -> Sum/1
  Step1/1 -> Sum/2
  Step2/1 -> Sum2/1
  Sum/1 -> Sum3/1
  Sum2/1 -> Sum3/2

== system simulation_Hippocampus_CDC/PDPD/HippCampus1/Subsystem ==
  In1 : Inport
  Demux : Demux  Outputs=[5 1 6]
  MATLAB Function : MATLAB Function  TreatAsAtomicUnit=on
  Mux : Mux  Inputs=3
  state : Outport
  wires:
  Demux/2 -> MATLAB Function/1(u)
  MATLAB Function/1(y) -> Mux/2
  In1/1 -> Demux/1
  Demux/3 -> Mux/3
  Demux/1 -> Mux/1
  Mux/1 -> state/1

== system simulation_Hippocampus_CDC/PDPD/HippCampus1/Subsystem1 ==
  u : Inport
  Integrator2 : Integrator
  Sqrt1 : Sqrt  SaturateOnIntegerOverflow=on
  norm1 : MATLAB Function  TreatAsAtomicUnit=on
  Out1 : Outport
  wires:
  norm1/1(y) -> Integrator2/1
  Sqrt1/1 -> Out1/1
  Integrator2/1 -> Sqrt1/1
  u/1 -> norm1/1(u)

== system simulation_Hippocampus_CDC/PDPD/HippCampus1/Subsystem4 ==
  u : Inport
  Demux : Demux
  Mux : Mux
  Subsystem : Subsystem
  Subsystem1 : Subsystem
  Subsystem2 : Subsystem
  Subsystem3 : Subsystem
  Out1 : Outport
  wires:
  Subsystem2/1(Out1) -> Mux/3
  Demux/4 -> Subsystem3/1(u)
  Demux/3 -> Subsystem2/1(u)
  Subsystem1/1(Out1) -> Mux/2
  Demux/2 -> Subsystem1/1(u)
  Subsystem3/1(Out1) -> Mux/4
  Demux/1 -> Subsystem/1(u)
  Subsystem/1(Out1) -> Mux/1
  Mux/1 -> Out1/1
  u/1 -> Demux/1

== system simulation_Hippocampus_CDC/Proposed controller/Disturbance: All derivatives1/disturbance2 ==
  Gain : Gain  Gain=[zeros(6,1);ones(6,1)]  Multiplication=Matrix(K*u)
  Step2 : Step  Time=50  After=0.5  SampleTime=0
  Step3 : Step  Time=55  After=-0.5  SampleTime=0
  Sum1 : Sum  Inputs=|++
  Out1 : Outport
  wires:
  Step2/1 -> Sum1/1
  Step3/1 -> Sum1/2
  Gain/1 -> Out1/1
  Sum1/1 -> Gain/1

== system simulation_Hippocampus_CDC/Proposed controller/Disturbance: All derivatives1/disturbance3 ==
  note: Subsystem
  a : Inport
  a1 : Inport  Port=2
  Constant : Constant  Value=10
  Constant2 : Constant  Value=10
  Constant3 : Constant  Value=45
  Constant4 : Constant  Value=20
  Gain : Gain  Gain=pi/180
  Gain1 : Gain  Gain=pi/180
  MATLAB Function : MATLAB Function  TreatAsAtomicUnit=on
  Mux : Mux  Inputs=3
  Subsystem1 : Subsystem
  d : Outport
  wires:
  Subsystem1/1(Out1) -> MATLAB Function/3(u_wave)
  Constant/1 -> MATLAB Function/5(u_un)
  Mux/1 -> MATLAB Function/4(u_c)
  MATLAB Function/1(d) -> d/1
  a1/1 -> MATLAB Function/1(p)
  a/1 -> MATLAB Function/2(a)
  Constant4/1 -> Mux/1
  Gain/1 -> Mux/2
  Gain1/1 -> Mux/3
  Constant3/1 -> Gain1/1
  Constant2/1 -> Gain/1

== system simulation_Hippocampus_CDC/Proposed controller/Disturbance: All derivatives1/old disturbance ==
  Gain : Gain  Gain=ones(12,1)  Multiplication=Matrix(K*u)
  Step : Step  Time=50  After=0.5  SampleTime=0
  Step1 : Step  Time=55  After=-0.5  SampleTime=0
  Step2 : Step  Time=100  After=0.5  SampleTime=0
  Step3 : Step  Time=105  After=-0.5  SampleTime=0
  Sum : Sum  Inputs=|++
  Sum2 : Sum  Inputs=|++
  Sum3 : Sum  Inputs=|++
  Out1 : Outport
  wires:
  Step/1 -> Sum/1
  Step1/1 -> Sum/2
  Gain/1 -> Out1/1
  Step2/1 -> Sum2/1
  Step3/1 -> Sum2/2
  Sum/1 -> Sum3/1
  Sum2/1 -> Sum3/2
  Sum3/1 -> Gain/1

== system simulation_Hippocampus_CDC/Proposed controller/HippCampus/Subsystem ==
  In1 : Inport
  Demux : Demux  Outputs=[5 1 1 1 4]
  MATLAB Function : MATLAB Function  TreatAsAtomicUnit=on
  Mux : Mux  Inputs=5
  state : Outport
  wires:
  Demux/2 -> MATLAB Function/1(u)
  MATLAB Function/1(y) -> Mux/2
  In1/1 -> Demux/1
  Demux/3 -> Mux/3
  Demux/1 -> Mux/1
  Mux/1 -> state/1
  Demux/5 -> Mux/5
  Demux/4 -> Mux/4

== system simulation_Hippocampus_CDC/Proposed controller/HippCampus/Subsystem1 ==
  u : Inport
  Integrator2 : Integrator
  Sqrt1 : Sqrt  SaturateOnIntegerOverflow=on
  norm1 : MATLAB Function  TreatAsAtomicUnit=on
  Out1 : Outport
  wires:
  norm1/1(y) -> Integrator2/1
  Sqrt1/1 -> Out1/1
  Integrator2/1 -> Sqrt1/1
  u/1 -> norm1/1(u)

== system simulation_Hippocampus_CDC/Proposed controller/HippCampus/Subsystem4 ==
  u : Inport
  Demux : Demux
  Mux : Mux
  Subsystem : Subsystem
  Subsystem1 : Subsystem
  Subsystem2 : Subsystem
  Subsystem3 : Subsystem
  Out1 : Outport
  wires:
  Subsystem2/1(Out1) -> Mux/3
  Demux/4 -> Subsystem3/1(u)
  Demux/3 -> Subsystem2/1(u)
  Subsystem1/1(Out1) -> Mux/2
  Demux/2 -> Subsystem1/1(u)
  Subsystem3/1(Out1) -> Mux/4
  Demux/1 -> Subsystem/1(u)
  Subsystem/1(Out1) -> Mux/1
  Mux/1 -> Out1/1
  u/1 -> Demux/1

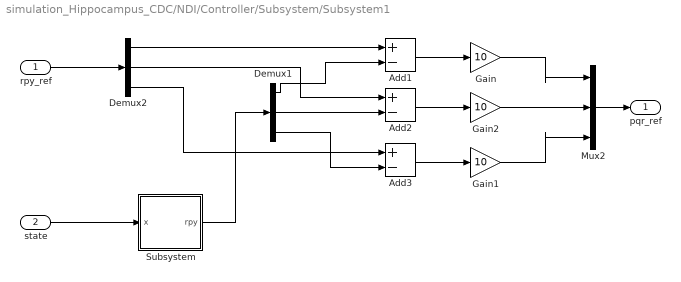
== system simulation_Hippocampus_CDC/NDI/Controller/Subsystem/Subsystem1 ==
  rpy_ref : Inport
  state : Inport  Port=2
  Add1 : Sum  Inputs=+-
  Add2 : Sum  Inputs=+-
  Add3 : Sum  Inputs=+-
  Demux1 : Demux  Outputs=3
  Demux2 : Demux  Outputs=3
  Gain : Gain  Gain=10
  Gain1 : Gain  Gain=10
  Gain2 : Gain  Gain=10
  Mux2 : Mux  Inputs=3
  Subsystem : Subsystem
  pqr_ref : Outport
  wires:
  state/1 -> Subsystem/1(x)
  Demux1/1 -> Add1/2
  Demux1/3 -> Add3/2
  Demux2/3 -> Add3/1
  Demux1/2 -> Add2/2
  Gain/1 -> Mux2/1
  Gain1/1 -> Mux2/3
  Add2/1 -> Gain2/1
  Gain2/1 -> Mux2/2
  Demux2/2 -> Add2/1
  Demux2/1 -> Add1/1
  Subsystem/1(rpy) -> Demux1/1
  rpy_ref/1 -> Demux2/1
  Add1/1 -> Gain/1
  Add3/1 -> Gain1/1
  Mux2/1 -> pqr_ref/1

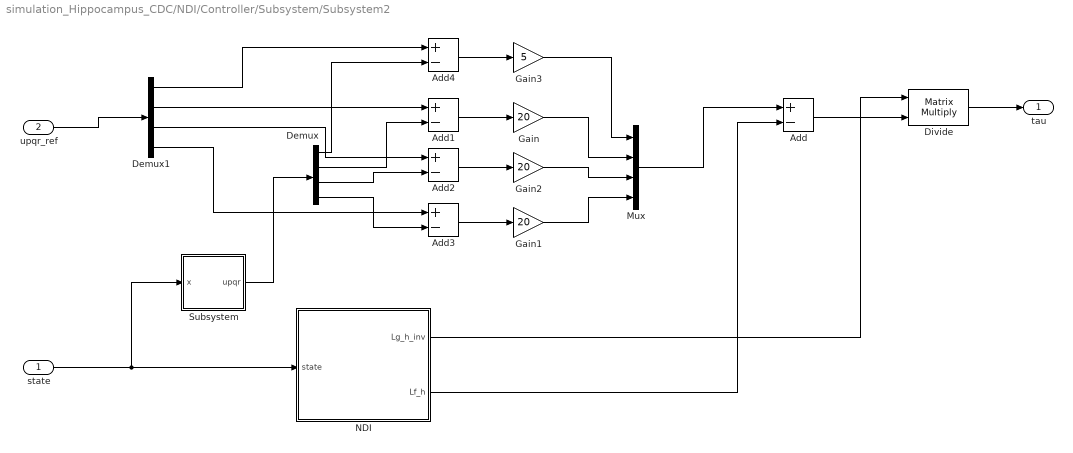
== system simulation_Hippocampus_CDC/NDI/Controller/Subsystem/Subsystem2 ==
  state : Inport
  upqr_ref : Inport  Port=2
  Add{,1..4} (5 alike) : Sum  Inputs=+-
  Demux : Demux
  Demux1 : Demux
  Divide : Product  Inputs=**  Multiplication=Matrix(*)
  Gain : Gain  Gain=20
  Gain1 : Gain  Gain=20
  Gain2 : Gain  Gain=20
  Gain3 : Gain  Gain=5
  Mux : Mux
  NDI : Subsystem
  Subsystem : Subsystem
  tau : Outport
  wires:
  Add1/1 -> Gain/1
  NDI/1(Lg_h_inv) -> Divide/1
  Mux/1 -> Add/1
  Add2/1 -> Gain2/1
  Add3/1 -> Gain1/1
  Divide/1 -> tau/1
  NDI/2(Lf_h) -> Add/2
  Add/1 -> Divide/2
  state/1 -> Subsystem/1(x), NDI/1(state)
  Subsystem/1(upqr) -> Demux/1
  Demux1/2 -> Add1/1
  Demux1/3 -> Add2/1
  Demux1/4 -> Add3/1
  upqr_ref/1 -> Demux1/1
  Gain1/1 -> Mux/4
  Gain2/1 -> Mux/3
  Gain/1 -> Mux/2
  Add4/1 -> Gain3/1
  Gain3/1 -> Mux/1
  Demux/1 -> Add4/2
  Demux/2 -> Add1/2
  Demux/3 -> Add2/2
  Demux/4 -> Add3/2
  Demux1/1 -> Add4/1

== system simulation_Hippocampus_CDC/NDI/Disturbance: All derivatives1/disturbance3/Subsystem ==
  Constant2 : Constant  Value=5
  Constant3 : Constant  Value=30
  Constant4 : Constant  Value=20
  Gain : Gain  Gain=pi/180
  Gain1 : Gain  Gain=pi/180
  Mux : Mux  Inputs=3
  Out1 : Outport
  wires:
  Constant2/1 -> Gain/1
  Constant3/1 -> Gain1/1
  Gain1/1 -> Mux/3
  Gain/1 -> Mux/2
  Mux/1 -> Out1/1
  Constant4/1 -> Mux/1

== system simulation_Hippocampus_CDC/NDI/Disturbance: All derivatives1/disturbance3/Subsystem1 ==
  Clock : Clock
  Mux1 : Mux  Inputs=3
  wave frenquency : Subsystem
  wave percentage : Subsystem
  Out1 : Outport
  wires:
  wave frenquency/1(Out1) -> Mux1/2
  Mux1/1 -> Out1/1
  wave percentage/1(Out1) -> Mux1/1
  Clock/1 -> Mux1/3

== system simulation_Hippocampus_CDC/NDI/HippCampus1/Subsystem4/Subsystem ==
  u : Inport
  Integrator2 : Integrator
  Sqrt1 : Sqrt  SaturateOnIntegerOverflow=on
  norm1 : MATLAB Function  TreatAsAtomicUnit=on
  Out1 : Outport
  wires:
  norm1/1(y) -> Integrator2/1
  Sqrt1/1 -> Out1/1
  Integrator2/1 -> Sqrt1/1
  u/1 -> norm1/1(u)

== system simulation_Hippocampus_CDC/NDI/HippCampus1/Subsystem4/Subsystem1 ==
  u : Inport
  Integrator2 : Integrator
  Sqrt1 : Sqrt  SaturateOnIntegerOverflow=on
  norm1 : MATLAB Function  TreatAsAtomicUnit=on
  Out1 : Outport
  wires:
  norm1/1(y) -> Integrator2/1
  Sqrt1/1 -> Out1/1
  Integrator2/1 -> Sqrt1/1
  u/1 -> norm1/1(u)

== system simulation_Hippocampus_CDC/NDI/HippCampus1/Subsystem4/Subsystem2 ==
  u : Inport
  Integrator2 : Integrator
  Sqrt1 : Sqrt  SaturateOnIntegerOverflow=on
  norm1 : MATLAB Function  TreatAsAtomicUnit=on
  Out1 : Outport
  wires:
  norm1/1(y) -> Integrator2/1
  Sqrt1/1 -> Out1/1
  Integrator2/1 -> Sqrt1/1
  u/1 -> norm1/1(u)

== system simulation_Hippocampus_CDC/NDI/HippCampus1/Subsystem4/Subsystem3 ==
  u : Inport
  Integrator2 : Integrator
  Sqrt1 : Sqrt  SaturateOnIntegerOverflow=on
  norm1 : MATLAB Function  TreatAsAtomicUnit=on
  Out1 : Outport
  wires:
  norm1/1(y) -> Integrator2/1
  Sqrt1/1 -> Out1/1
  Integrator2/1 -> Sqrt1/1
  u/1 -> norm1/1(u)

== system simulation_Hippocampus_CDC/PDPD/Disturbance: All derivatives1/disturbance3/Subsystem1 ==
  Clock : Clock
  Mux1 : Mux  Inputs=3
  wave frenquency : Subsystem
  wave percentage : Subsystem
  Out1 : Outport
  wires:
  wave frenquency/1(Out1) -> Mux1/2
  Mux1/1 -> Out1/1
  wave percentage/1(Out1) -> Mux1/1
  Clock/1 -> Mux1/3

== system simulation_Hippocampus_CDC/PDPD/HippCampus1/Subsystem4/Subsystem ==
  u : Inport
  Integrator2 : Integrator
  Sqrt1 : Sqrt  SaturateOnIntegerOverflow=on
  norm1 : MATLAB Function  TreatAsAtomicUnit=on
  Out1 : Outport
  wires:
  norm1/1(y) -> Integrator2/1
  Sqrt1/1 -> Out1/1
  Integrator2/1 -> Sqrt1/1
  u/1 -> norm1/1(u)

== system simulation_Hippocampus_CDC/PDPD/HippCampus1/Subsystem4/Subsystem1 ==
  u : Inport
  Integrator2 : Integrator
  Sqrt1 : Sqrt  SaturateOnIntegerOverflow=on
  norm1 : MATLAB Function  TreatAsAtomicUnit=on
  Out1 : Outport
  wires:
  norm1/1(y) -> Integrator2/1
  Sqrt1/1 -> Out1/1
  Integrator2/1 -> Sqrt1/1
  u/1 -> norm1/1(u)

== system simulation_Hippocampus_CDC/PDPD/HippCampus1/Subsystem4/Subsystem2 ==
  u : Inport
  Integrator2 : Integrator
  Sqrt1 : Sqrt  SaturateOnIntegerOverflow=on
  norm1 : MATLAB Function  TreatAsAtomicUnit=on
  Out1 : Outport
  wires:
  norm1/1(y) -> Integrator2/1
  Sqrt1/1 -> Out1/1
  Integrator2/1 -> Sqrt1/1
  u/1 -> norm1/1(u)

== system simulation_Hippocampus_CDC/PDPD/HippCampus1/Subsystem4/Subsystem3 ==
  u : Inport
  Integrator2 : Integrator
  Sqrt1 : Sqrt  SaturateOnIntegerOverflow=on
  norm1 : MATLAB Function  TreatAsAtomicUnit=on
  Out1 : Outport
  wires:
  norm1/1(y) -> Integrator2/1
  Sqrt1/1 -> Out1/1
  Integrator2/1 -> Sqrt1/1
  u/1 -> norm1/1(u)

== system simulation_Hippocampus_CDC/Proposed controller/Disturbance: All derivatives1/disturbance3/Subsystem1 ==
  Clock : Clock
  Mux1 : Mux  Inputs=3
  wave frenquency : Subsystem
  wave percentage : Subsystem
  Out1 : Outport
  wires:
  wave frenquency/1(Out1) -> Mux1/2
  Mux1/1 -> Out1/1
  wave percentage/1(Out1) -> Mux1/1
  Clock/1 -> Mux1/3

== system simulation_Hippocampus_CDC/Proposed controller/HippCampus/Subsystem4/Subsystem ==
  u : Inport
  Integrator2 : Integrator
  Sqrt1 : Sqrt  SaturateOnIntegerOverflow=on
  norm1 : MATLAB Function  TreatAsAtomicUnit=on
  Out1 : Outport
  wires:
  norm1/1(y) -> Integrator2/1
  Sqrt1/1 -> Out1/1
  Integrator2/1 -> Sqrt1/1
  u/1 -> norm1/1(u)

== system simulation_Hippocampus_CDC/Proposed controller/HippCampus/Subsystem4/Subsystem1 ==
  u : Inport
  Integrator2 : Integrator
  Sqrt1 : Sqrt  SaturateOnIntegerOverflow=on
  norm1 : MATLAB Function  TreatAsAtomicUnit=on
  Out1 : Outport
  wires:
  norm1/1(y) -> Integrator2/1
  Sqrt1/1 -> Out1/1
  Integrator2/1 -> Sqrt1/1
  u/1 -> norm1/1(u)

== system simulation_Hippocampus_CDC/Proposed controller/HippCampus/Subsystem4/Subsystem2 ==
  u : Inport
  Integrator2 : Integrator
  Sqrt1 : Sqrt  SaturateOnIntegerOverflow=on
  norm1 : MATLAB Function  TreatAsAtomicUnit=on
  Out1 : Outport
  wires:
  norm1/1(y) -> Integrator2/1
  Sqrt1/1 -> Out1/1
  Integrator2/1 -> Sqrt1/1
  u/1 -> norm1/1(u)

== system simulation_Hippocampus_CDC/Proposed controller/HippCampus/Subsystem4/Subsystem3 ==
  u : Inport
  Integrator2 : Integrator
  Sqrt1 : Sqrt  SaturateOnIntegerOverflow=on
  norm1 : MATLAB Function  TreatAsAtomicUnit=on
  Out1 : Outport
  wires:
  norm1/1(y) -> Integrator2/1
  Sqrt1/1 -> Out1/1
  Integrator2/1 -> Sqrt1/1
  u/1 -> norm1/1(u)

== system simulation_Hippocampus_CDC/NDI/Controller/Subsystem/Subsystem1/Subsystem ==
  x : Inport
  Demux : Demux  Outputs=12
  Mux : Mux  Inputs=3
  Terminator{,1..8} (9 alike) : Terminator
  rpy : Outport
  wires:
  x/1 -> Demux/1
  Demux/6 -> Mux/3
  Mux/1 -> rpy/1
  Demux/5 -> Mux/2
  Demux/4 -> Mux/1
  Demux/1 -> Terminator/1
  Demux/2 -> Terminator1/1
  Demux/3 -> Terminator2/1
  Demux/7 -> Terminator3/1
  Demux/9 -> Terminator5/1
  Demux/10 -> Terminator6/1
  Demux/11 -> Terminator7/1
  Demux/12 -> Terminator8/1
  Demux/8 -> Terminator4/1

== system simulation_Hippocampus_CDC/NDI/Controller/Subsystem/Subsystem2/NDI ==
  state : Inport
  Demux : Demux  Outputs=12
  Demux1 : Demux  Outputs=12
  Lf : MATLAB Function  TreatAsAtomicUnit=on
  Lg : MATLAB Function  TreatAsAtomicUnit=on
  Lg_h_inv : Outport
  Lf_h : Outport  Port=2
  wires:
  Demux/6 -> Lg/6(psi)
  Demux1/11 -> Lf/11(q)
  Demux/4 -> Lg/4(phi)
  Demux1/5 -> Lf/5(theta)
  Demux1/6 -> Lf/6(psi)
  Demux/2 -> Lg/2(y)
  Demux/7 -> Lg/7(u)
  Demux1/2 -> Lf/2(y)
  Demux1/1 -> Lf/1(x)
  state/1 -> Demux/1, Demux1/1
  Demux1/4 -> Lf/4(phi)
  Demux1/7 -> Lf/7(u)
  Demux/1 -> Lg/1(x)
  Demux/12 -> Lg/12(r)
  Demux/5 -> Lg/5(theta)
  Demux/8 -> Lg/8(v)
  Lf/1(Lf_h) -> Lf_h/1
  Demux/3 -> Lg/3(z)
  Demux/11 -> Lg/11(q)
  Demux1/8 -> Lf/8(v)
  Demux1/3 -> Lf/3(z)
  Demux/10 -> Lg/10(p)
  Demux1/12 -> Lf/12(r)
  Lg/1(Lg_h_inv) -> Lg_h_inv/1
  Demux1/9 -> Lf/9(w)
  Demux1/10 -> Lf/10(p)
  Demux/9 -> Lg/9(w)

== system simulation_Hippocampus_CDC/NDI/Controller/Subsystem/Subsystem2/Subsystem ==
  x : Inport
  Demux : Demux  Outputs=12
  Mux : Mux
  Terminator{1..8} (8 alike) : Terminator
  upqr : Outport
  wires:
  x/1 -> Demux/1
  Mux/1 -> upqr/1
  Demux/12 -> Mux/4
  Demux/11 -> Mux/3
  Demux/10 -> Mux/2
  Demux/7 -> Mux/1
  Demux/1 -> Terminator4/1
  Demux/2 -> Terminator1/1
  Demux/3 -> Terminator2/1
  Demux/4 -> Terminator3/1
  Demux/5 -> Terminator5/1
  Demux/6 -> Terminator6/1
  Demux/8 -> Terminator7/1
  Demux/9 -> Terminator8/1

== system simulation_Hippocampus_CDC/NDI/Disturbance: All derivatives1/disturbance3/Subsystem1/wave frenquency ==
  Constant2 : Constant
  Constant3 : Constant  Value=1.1
  Constant4 : Constant  Value=1.2
  Constant5 : Constant  Value=0.5
  Constant6 : Constant  Value=0.6
  Constant7 : Constant  Value=0.7
  Mux : Mux  Inputs=6
  Out1 : Outport
  wires:
  Constant3/1 -> Mux/2
  Constant2/1 -> Mux/1
  Constant4/1 -> Mux/3
  Constant7/1 -> Mux/6
  Mux/1 -> Out1/1
  Constant5/1 -> Mux/4
  Constant6/1 -> Mux/5

== system simulation_Hippocampus_CDC/NDI/Disturbance: All derivatives1/disturbance3/Subsystem1/wave percentage ==
  Constant{2..7} (6 alike) : Constant  Value=0
  Mux : Mux  Inputs=6
  Out1 : Outport
  wires:
  Constant3/1 -> Mux/2
  Constant2/1 -> Mux/1
  Constant4/1 -> Mux/3
  Constant7/1 -> Mux/6
  Mux/1 -> Out1/1
  Constant5/1 -> Mux/4
  Constant6/1 -> Mux/5

== system simulation_Hippocampus_CDC/PDPD/Disturbance: All derivatives1/disturbance3/Subsystem1/wave frenquency ==
  Constant2 : Constant
  Constant3 : Constant  Value=1.1
  Constant4 : Constant  Value=1.2
  Constant5 : Constant  Value=0.5
  Constant6 : Constant  Value=0.6
  Constant7 : Constant  Value=0.7
  Mux : Mux  Inputs=6
  Out1 : Outport
  wires:
  Constant3/1 -> Mux/2
  Constant2/1 -> Mux/1
  Constant4/1 -> Mux/3
  Constant7/1 -> Mux/6
  Mux/1 -> Out1/1
  Constant5/1 -> Mux/4
  Constant6/1 -> Mux/5

== system simulation_Hippocampus_CDC/PDPD/Disturbance: All derivatives1/disturbance3/Subsystem1/wave percentage ==
  Constant{2..7} (6 alike) : Constant  Value=0
  Mux : Mux  Inputs=6
  Out1 : Outport
  wires:
  Constant3/1 -> Mux/2
  Constant2/1 -> Mux/1
  Constant4/1 -> Mux/3
  Constant7/1 -> Mux/6
  Mux/1 -> Out1/1
  Constant5/1 -> Mux/4
  Constant6/1 -> Mux/5

== system simulation_Hippocampus_CDC/Proposed controller/Disturbance: All derivatives1/disturbance3/Subsystem1/wave frenquency ==
  Constant2 : Constant
  Constant3 : Constant  Value=1.1
  Constant4 : Constant  Value=1.2
  Constant5 : Constant  Value=0.5
  Constant6 : Constant  Value=0.6
  Constant7 : Constant  Value=0.7
  Mux : Mux  Inputs=6
  Out1 : Outport
  wires:
  Constant3/1 -> Mux/2
  Constant2/1 -> Mux/1
  Constant4/1 -> Mux/3
  Constant7/1 -> Mux/6
  Mux/1 -> Out1/1
  Constant5/1 -> Mux/4
  Constant6/1 -> Mux/5

== system simulation_Hippocampus_CDC/Proposed controller/Disturbance: All derivatives1/disturbance3/Subsystem1/wave percentage ==
  Constant{2..7} (6 alike) : Constant  Value=0
  Mux : Mux  Inputs=6
  Out1 : Outport
  wires:
  Constant3/1 -> Mux/2
  Constant2/1 -> Mux/1
  Constant4/1 -> Mux/3
  Constant7/1 -> Mux/6
  Mux/1 -> Out1/1
  Constant5/1 -> Mux/4
  Constant6/1 -> Mux/5

== matlab function simulation_Hippocampus_CDC/PDPD/HippCampus1/Subsystem/MATLAB Function ==
  data: u input; y output
function y = fcn(u)
y =  wrapToPi(u);

== matlab function simulation_Hippocampus_CDC/PDPD/HippCampus1/sat2 ==
  data: u input; u_sat output; omega output
function [u_sat, omega] = fcn(u)
  %  u_sat=u;
    h     = 0.0481;   % [m] Distance of rotors to HippoCampus center
    Cd    = 0.0024;   % Coefficient of drag for the rotors
    tlim  = 3;        % Maximal torque of the motors 

    Q = [1,1,1,1;-Cd,Cd,-Cd,Cd;-h,-h,h,h;h,-h,-h,h];
    Qinv = inv(Q);

    % Transform into rotor space
    omega = Qinv*u;

    % Calculate utilization of each rotor
    util  = abs(omega/tlim);

    % Saturate torque at max utilization
    omega = omega ./ max(util, 1);    

    %Transform back into body frame
   u_sat = Q * omega;
end

== matlab function simulation_Hippocampus_CDC/PDPD/norm ==
  data: u input; y output
function y  = fcn(u)
y=norm(u)^2;
end

== matlab function simulation_Hippocampus_CDC/PDPD/Disturbance: All derivatives1/disturbance3/MATLAB Function ==
  data: p input; a input; d output; u_wave input; u_c input; u_un input
%% wind disturbance, wave disturbance, ocean currents and modeling uncertainties(Fossen 2011)
%for AUV, we can neglect the wind disturbance
%wave disturbance is in R^6
%Ocean Currents are related to the hydrodynamic terms. Here we consider
%them as the friction forces 
%modeling uncertainties can be assumed as constant terms
%assume all disturbances are constant
function d = fcn(p,a,u_wave, u_c,u_un)
%a: attitude states
%u_wave: parameters of u_wave
%u_c ocean currents percentage
%u_un uncertainty percentage
%ocean currents
phi=a(1);
theta=a(2);
psi = a(3);
V = u_c(1)/100*4.724; % 0<V<4.724
theta_c=u_c(2);
psi_c = u_c(3);
 R = [  cos(psi)*cos(theta)  cos(psi)*sin(theta)*sin(phi)-sin(psi)*cos(phi)  cos(psi)*cos(phi)*sin(theta)+sin(psi)*sin(phi) ;
           sin(psi)*cos(theta)  sin(psi)*sin(theta)*sin(phi)+cos(psi)*cos(phi)  sin(psi)*cos(phi)*sin(theta)-cos(psi)*sin(phi) ;
          -sin(theta)           cos(theta)*sin(phi)                             cos(theta)*cos(phi)                            ];
uc=[V*cos(theta_c)*cos(psi_c);V*sin(psi_c);V*sin(theta_c)*cos(psi_c)];
f_c=R*uc;
d_c=[f_c;zeros(3,1)];

%wave disturbance
k1=u_wave(1:6); %amplitude 
k2 = u_wave(7:12); %frequency 
time=u_wave(13);
d_w = [k1(1)/100*4.724*sin(k2(1)*time);k1(2)/100*4.724*sin(k2(2)*time);k1(3)/100*4.724*sin(k2(3)*time);
    k1(4)/100*6.841*sin(k2(4)*time);k1(5)/100*28.55*sin(k2(5)*time);k1(6)/100*28.55*sin(k2(6)*time)];
%model uncertainties
%u_un uncertainty percentage
d_u=u_un/100*[4.724;0;0;6.841;28.55;28.55];

x=p(1);
y=p(2);
z=p(3);
if y>2 && y<2.5 || y<-2 && y>-2.5
    tau_d=d_c+d_w+d_u;
else
    tau_d=zeros(6,1);
end
    
d=[zeros(6,1);tau_d];

== matlab function simulation_Hippocampus_CDC/NDI/Controller/MATLAB Function ==
  data: theta_des input; theta_des output; x input
function theta_des = fcn(theta_des, x)
yaw = x(6);
yaw_des = theta_des(3);
e_yaw = yaw_des-yaw;

% jump from -pi to +pi
if (e_yaw > pi)
    yaw_des = yaw_des - 2*pi;
% jump from +pi to -pi
elseif (-e_yaw > pi)
    yaw_des = yaw_des + 2*pi;
end
theta_des(3) = yaw_des;

== matlab function simulation_Hippocampus_CDC/Proposed controller/norm ==
  data: u input; y output
function y  = fcn(u)
y=norm(u)^2;
end
